simulink subsystem "Hardware_Interface"  (R2022b)
settings: Solver=VariableStepAuto  StartTime=0.0  StopTime=10.0  RelTol=1e-3
undefined symbols (not defined in the file): AS5600, INA219
libraries: arduinolib x10, hdlsllib x2
settings Model: Creator=gotta  LastModifiedBy=gotta

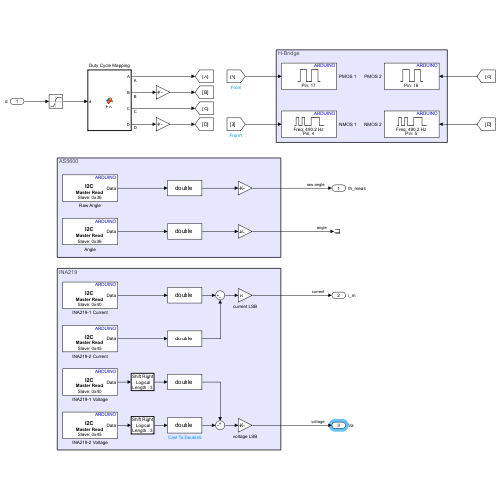
[thumbnail: Simulink's stored preview of the top-level diagram]
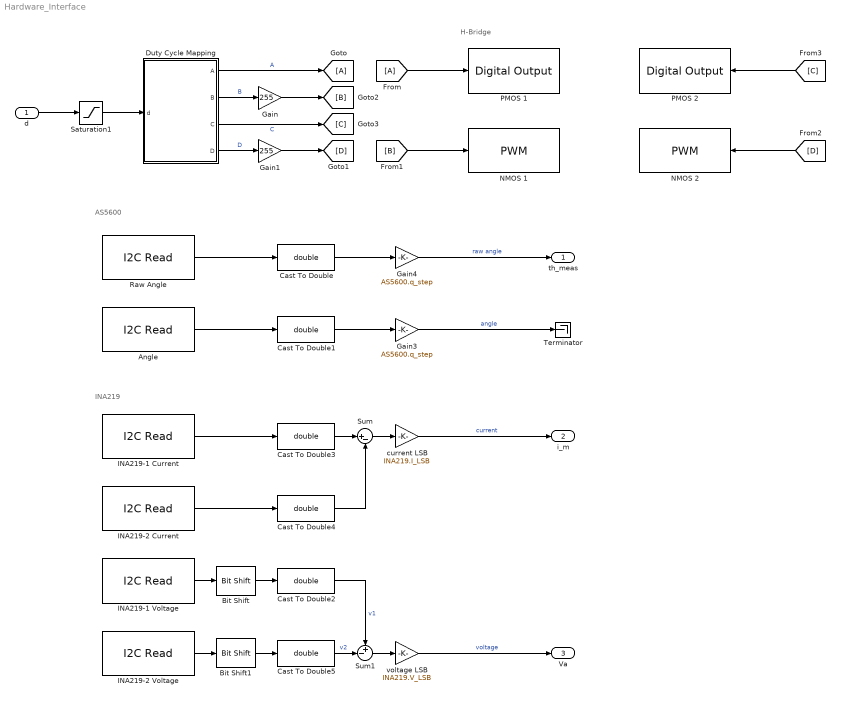
== system Hardware_Interface ==
  note: INA219
  note: AS5600
  note: H-Bridge
  d : Inport
  Angle : arduinolib/I2C Read  I2CModule=0  Mode=Master  SlaveAddress=AS5600.DEV_ADDR  SlaveByteOrder=BigEndian  Direction=Receiver  RegisterAddressMode=on  RegisterAddress=AS5600.ANGLE_ADDR  SlaveDataType=int16  DataLength=1  NoAck=off  RepeatedStart=off  OutputStatus=off  blockPlatform=ARDUINO  SampleTime=1e-3
  Bit Shift : hdlsllib/Logic and Bit Operations/Bit Shift  mode=Shift Right Logical  N=3
  Bit Shift1 : hdlsllib/Logic and Bit Operations/Bit Shift  mode=Shift Right Logical  N=3
  Cast To Double{,1..5} (6 alike) : DataTypeConversion  OutDataTypeStr=double  SaturateOnIntegerOverflow=off  RndMeth=Floor
  Duty Cycle Mapping : MATLAB Function  TreatAsAtomicUnit=on
  From : From
  Gain : Gain  Gain=255
  Gain1 : Gain  Gain=255
  Gain3 : Gain  Gain=AS5600.q_step
  Gain4 : Gain  Gain=AS5600.q_step
  Goto : Goto
  INA219-1 Current : arduinolib/I2C Read  I2CModule=0  Mode=Master  SlaveAddress=INA219.DEV1_ADDR  SlaveByteOrder=BigEndian  Direction=Receiver  RegisterAddressMode=on  RegisterAddress=INA219.I_ADDR  SlaveDataType=int16  DataLength=1  NoAck=off  RepeatedStart=off  OutputStatus=off  blockPlatform=ARDUINO  SampleTime=1e-3
  INA219-1 Voltage : arduinolib/I2C Read  I2CModule=0  Mode=Master  SlaveAddress=INA219.DEV1_ADDR  SlaveByteOrder=BigEndian  Direction=Receiver  RegisterAddressMode=on  RegisterAddress=INA219.BusV_ADDR  SlaveDataType=uint16  DataLength=1  NoAck=off  RepeatedStart=off  OutputStatus=off  blockPlatform=ARDUINO  SampleTime=1e-3
  INA219-2 Current : arduinolib/I2C Read  I2CModule=0  Mode=Master  SlaveAddress=INA219.DEV2_ADDR  SlaveByteOrder=BigEndian  Direction=Receiver  RegisterAddressMode=on  RegisterAddress=INA219.I_ADDR  SlaveDataType=int16  DataLength=1  NoAck=off  RepeatedStart=off  OutputStatus=off  blockPlatform=ARDUINO  SampleTime=1e-3
  INA219-2 Voltage : arduinolib/I2C Read  I2CModule=0  Mode=Master  SlaveAddress=INA219.DEV2_ADDR  SlaveByteOrder=BigEndian  Direction=Receiver  RegisterAddressMode=on  RegisterAddress=INA219.BusV_ADDR  SlaveDataType=uint16  DataLength=1  NoAck=off  RepeatedStart=off  OutputStatus=off  blockPlatform=ARDUINO  SampleTime=1e-3
  NMOS 1 : arduinolib/PWM  pinNumber=4  frequencyType=Specify  desiredFrequency=2e4  achievableFrequency=20000
  NMOS 2 : arduinolib/PWM  pinNumber=5  frequencyType=Specify  desiredFrequency=2e4  achievableFrequency=20000
  PMOS 1 : arduinolib/Digital Output  pinNumber=17  Direction=output  blockPlatform=arduino
  PMOS 2 : arduinolib/Digital Output  pinNumber=16  Direction=output  blockPlatform=arduino
  Raw Angle : arduinolib/I2C Read  I2CModule=0  Mode=Master  SlaveAddress=AS5600.DEV_ADDR  SlaveByteOrder=BigEndian  Direction=Receiver  RegisterAddressMode=on  RegisterAddress=AS5600.RANGLE_ADDR  SlaveDataType=int16  DataLength=1  NoAck=off  RepeatedStart=off  OutputStatus=off  blockPlatform=ARDUINO  SampleTime=1e-3
  Saturation1 : Saturate  UpperLimit=1  LowerLimit=-1
  Sum : Sum  Inputs=|+-
  Sum1 : Sum  Inputs=+-|
  Terminator : Terminator
  current LSB : Gain  Gain=INA219.I_LSB
  voltage LSB : Gain  Gain=INA219.V_LSB
  th_meas : Outport
  i_m : Outport  Port=2
  Va : Outport  Port=3
  wires:
  d/1 -> Saturation1/1
  Duty Cycle Mapping/4(D) -> Gain1/1  "D"
  Gain1/1 -> [D]
  Duty Cycle Mapping/3(C) -> [C]  "C"
  Saturation1/1 -> Duty Cycle Mapping/1(d)
  Duty Cycle Mapping/2(B) -> Gain/1  "B"
  Duty Cycle Mapping/1(A) -> Goto/1  "A"
  Gain/1 -> [B]
  From/1 -> PMOS 1/1
  [C] -> PMOS 2/1
  [B] -> NMOS 1/1
  [D] -> NMOS 2/1
  Sum1/1 -> voltage LSB/1
  current LSB/1 -> i_m/1  "current"
  Sum/1 -> current LSB/1
  Gain4/1 -> th_meas/1  "raw angle"
  Cast To Double4/1 -> Sum/2
  Cast To Double3/1 -> Sum/1
  Cast To Double2/1 -> Sum1/1  "v1"
  Cast To Double5/1 -> Sum1/2  "v2"
  Gain3/1 -> Terminator/1  "angle"
  Cast To Double1/1 -> Gain3/1
  Angle/1 -> Cast To Double1/1
  Raw Angle/1 -> Cast To Double/1
  Cast To Double/1 -> Gain4/1
  Bit Shift/1 -> Cast To Double2/1
  INA219-1 Voltage/1 -> Bit Shift/1
  INA219-1 Current/1 -> Cast To Double3/1
  Bit Shift1/1 -> Cast To Double5/1
  INA219-2 Voltage/1 -> Bit Shift1/1
  INA219-2 Current/1 -> Cast To Double4/1
  voltage LSB/1 -> Va/1  "voltage"

== matlab function Hardware_Interface/Duty Cycle Mapping ==
  data: d input; A output; B output; C output; D output
function [A, B, C, D]= fcn(d)

direction = sign(d);
amplitude = abs(d);

A = 0;
B = 0;
C = 0;
D = 0;

if direction > 0
    % Act on A, D
    A = 1;
    B = 0;
    C = 0;
    D = amplitude;
elseif direction < 0
    % Act on B, C
    A = 0;
    B = amplitude;
    C = 1;
    D = 0;
end
